simulink model "Second_order_simulink"  (R2020b)
settings: Solver=VariableStepAuto  StartTime=0.0  StopTime=100  RelTol=1e-3
settings Model: Creator=99003785  LastModifiedBy=99003729

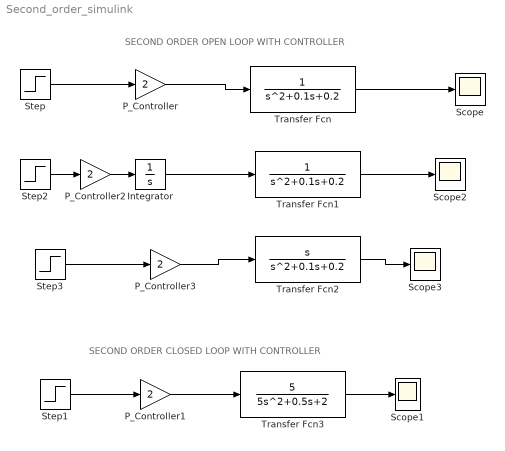
== system Second_order_simulink ==
  note: SECOND ORDER OPEN LOOP WITH CONTROLLER
  note: SECOND ORDER CLOSED LOOP WITH CONTROLLER
  Integrator : Integrator
  P_Controller{,1..3} (4 alike) : Gain  Gain=2
  Scope{,1..3} (4 alike) : Scope
  Step{,1..3} (4 alike) : Step  SampleTime=0
  Transfer Fcn : TransferFcn  Denominator=[1 0.1 0.2]
  Transfer Fcn1 : TransferFcn  Denominator=[1 0.1 0.2]
  Transfer Fcn2 : TransferFcn  Numerator=[1 0]  Denominator=[1 0.1 0.2]
  Transfer Fcn3 : TransferFcn  Numerator=[5]  Denominator=[5 0.5 2]
  wires:
  Step2/1 -> P_Controller2/1
  P_Controller2/1 -> Integrator/1
  Step3/1 -> P_Controller3/1
  Step1/1 -> P_Controller1/1
  Transfer Fcn/1 -> Scope/1
  Step/1 -> P_Controller/1
  P_Controller/1 -> Transfer Fcn/1
  Transfer Fcn1/1 -> Scope2/1
  Integrator/1 -> Transfer Fcn1/1
  P_Controller3/1 -> Transfer Fcn2/1
  Transfer Fcn2/1 -> Scope3/1
  Transfer Fcn3/1 -> Scope1/1
  P_Controller1/1 -> Transfer Fcn3/1
